simulink model "full_observer"  (R2020b)
settings: Solver=FixedStepAuto  StartTime=0.0  StopTime=20  FixedStep=0.01  RelTol=1e-3
values from neighbouring files (symbols this model uses):
  G = -J_RH*(M_M*L/2+M*l)*(J_RH+N^2*J_m+j)*g    (= -0.22537747671)    [aaaaaaaaaaaaaaaaaaaaaaaaa.m]    (also in disturb_estimation.m = -0.0465293382657; full_obs2.m = -0.0465293382657; fuulll_feedback.m = -0.0465293382657; reduced_observre_2.m = -0.0465293382657)
  H = -N*K_m*J_RH    (= -0.00759948)    [aaaaaaaaaaaaaaaaaaaaaaaaa.m]    (also in disturb_estimation.m = -0.00486576; full_obs2.m = -0.00486576; fuulll_feedback.m = -0.00486576; reduced_observre_2.m = -0.00486576)
  k1 = K(1)    [disturb_estimation.m]    (also in full_obs2.m; fuulll_feedback.m; reduced_observre_2.m)
  k2 = K(2)    [disturb_estimation.m]    (also in full_obs2.m; fuulll_feedback.m; reduced_observre_2.m)
  k3 = K(3)    [disturb_estimation.m]    (also in full_obs2.m; fuulll_feedback.m; reduced_observre_2.m)
  k4 = K(4)    [disturb_estimation.m]    (also in full_obs2.m; fuulll_feedback.m; reduced_observre_2.m)
  K_m = 0.0109    [aaaaaaaaaaaaaaaaaaaaaaaaa.m]    (also in disturb_estimation.m; full_obs2.m; fuulll_feedback.m; reduced_observre_2.m)
  l1 = L(1)    [disturb_estimation.m]    (also in full (2).m = 0.06; full_obs2.m)
  l2 = L(2)    [disturb_estimation.m]    (also in full (2).m = 0.6329; full_obs2.m)
  l3 = L(3)    [disturb_estimation.m]    (also in full (2).m = 0.3; full_obs2.m)
  l4 = L(4)    [disturb_estimation.m]    (also in full (2).m = 0.0875; full_obs2.m)
  l5 = L(5)    [disturb_estimation.m]    (also in full (2).m = 0.0254; full_obs2.m)
  L_m = 0.145    [aaaaaaaaaaaaaaaaaaaaaaaaa.m]    (also in disturb_estimation.m; full_obs2.m; fuulll_feedback.m; reduced_observre_2.m)
  N = 14    [aaaaaaaaaaaaaaaaaaaaaaaaa.m]    (also in disturb_estimation.m = 3; full (2).m = -1.06605676; full_obs2.m = 3; fuulll_feedback.m = 3)
  R_m = 1.6    [aaaaaaaaaaaaaaaaaaaaaaaaa.m]    (also in disturb_estimation.m; full_obs2.m; fuulll_feedback.m; reduced_observre_2.m)
  T = (M_M*L/2+M*l)*(J_RH+N^2*J_m+j)*g    (= 4.52565214276)    [aaaaaaaaaaaaaaaaaaaaaaaaa.m]    (also in disturb_estimation.m = 0.312697165764; full (2).m = [T1;T2;T3;T4;T5;T6;T7]; full_obs2.m = 0.312697165764; fuulll_feedback.m = 0.312697165764)
  W = (J_M+M*l^2)*(J_RH+N^2*J_m+j)-(J_RH)^2    (= 0.0397505665657)    [aaaaaaaaaaaaaaaaaaaaaaaaa.m]    (also in disturb_estimation.m = -0.0192235420783; full (2).m = blkdiag(W_1,W_2,W_3,W_4,W_5,W_6,W_7); full_obs2.m = -0.0192235420783; fuulll_feedback.m = -0.0192235420783)
  Z = (J_M+M*l^2)*(J_RH+N^2*J_m+j)^2-J_RH^2*(J_RH+N^2*J_m+j)    (= 0.251295170273)    [aaaaaaaaaaaaaaaaaaaaaaaaa.m]    (also in disturb_estimation.m = -0.00839686182665; full_obs2.m = -0.00839686182665; fuulll_feedback.m = -0.00839686182665; reduced_observre_2.m = -0.00839686182665)
settings Model: Creator=A family  LastModifiedBy=A family

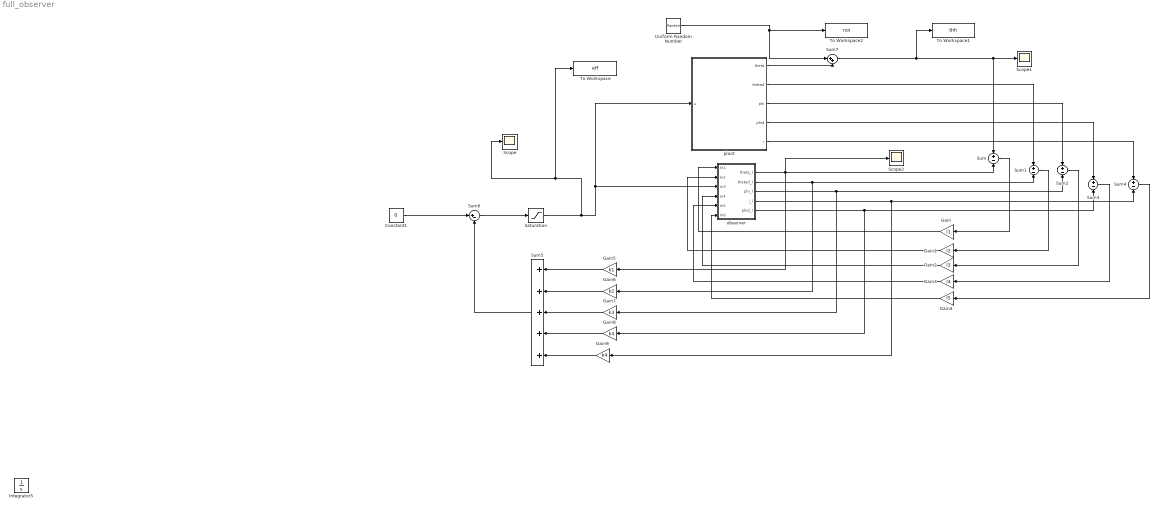
== system full_observer ==
  Constant1 : Constant  Value=0
  Gain : Gain  Gain=l1
  Gain1 : Gain  Gain=l2
  Gain2 : Gain  Gain=l3
  Gain3 : Gain  Gain=l4
  Gain4 : Gain  Gain=l5
  Gain5 : Gain  Gain=k1
  Gain6 : Gain  Gain=k2
  Gain7 : Gain  Gain=k3
  Gain8 : Gain  Gain=k4
  Gain9 : Gain  Gain=k4
  Integrator5 : Integrator
  Saturation : Saturate  UpperLimit=6  LowerLimit=-6
  Scope : Scope
  Scope1 : Scope
  Scope2 : Scope
  Sum{,1..4} (5 alike) : Sum  Inputs=+-
  Sum5 : Sum  Inputs=+++++
  Sum6 : Sum  Inputs=|+-
  Sum7 : Sum  Inputs=|++
  To Workspace : ToWorkspace  VariableName=eff  SampleTime=-1
  To Workspace1 : ToWorkspace  VariableName=thh  SampleTime=-1
  To Workspace2 : ToWorkspace  VariableName=noi  SampleTime=-1
  Uniform Random Number : UniformRandomNumber  Minimum=-0.1  Maximum=0.1  SampleTime=0.01
  observer : Subsystem
  plant : Subsystem
  wires:
  plant/2(thetad) -> Sum1/1
  plant/3(phi) -> Sum2/1
  plant/4(phid) -> Sum3/1
  plant/5(i) -> Sum4/1
  Sum/1 -> Gain/1
  Sum1/1 -> Gain1/1
  Sum2/1 -> Gain2/1
  Sum3/1 -> Gain3/1
  Sum4/1 -> Gain4/1
  Gain/1 -> observer/1(In1)
  Gain1/1 -> observer/2(In2)
  Gain2/1 -> observer/4(In4)
  Gain3/1 -> observer/5(In5)
  Gain4/1 -> observer/6(In6)
  observer/1(theta_l) -> Scope2/1, Gain5/1, Sum/2
  observer/2(thetad_l) -> Gain6/1, Sum1/2
  observer/3(phi_l) -> Gain7/1, Sum2/2
  observer/4(i_l) -> Gain9/1, Sum4/2
  observer/5(phid_l) -> Gain8/1, Sum3/2
  Gain5/1 -> Sum5/1
  Gain6/1 -> Sum5/2
  Gain7/1 -> Sum5/3
  Gain8/1 -> Sum5/4
  Gain9/1 -> Sum5/5
  Sum5/1 -> Sum6/2
  Constant1/1 -> Sum6/1
  Saturation/1 -> To Workspace/1, Scope/1, plant/1(u), observer/3(In3)
  Sum6/1 -> Saturation/1
  Uniform Random Number/1 -> To Workspace2/1, Sum7/1
  plant/1(theta) -> Sum7/2
  Sum7/1 -> To Workspace1/1, Sum/1, Scope1/1

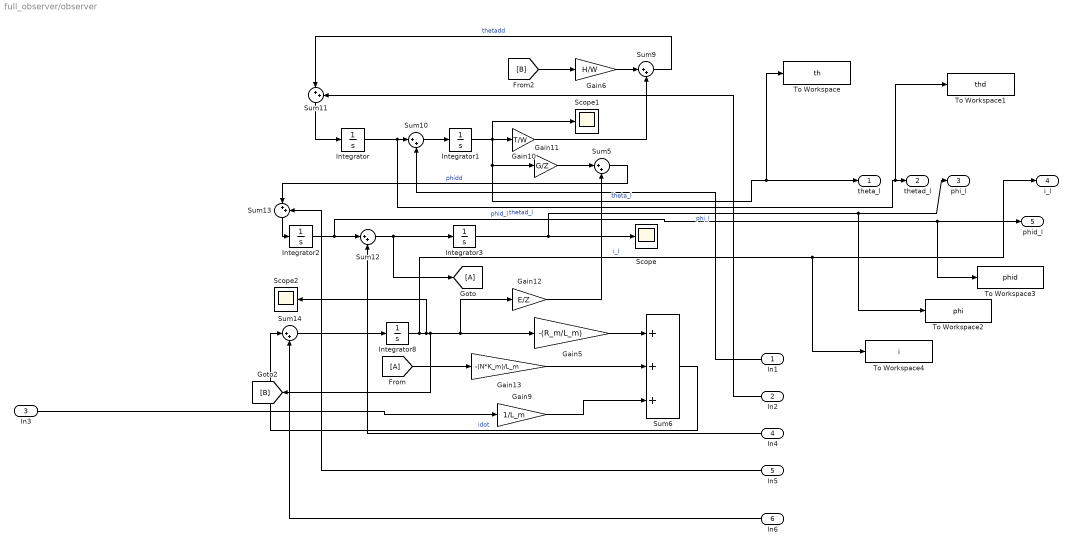
== system full_observer/observer ==
  In1 : Inport
  In2 : Inport  Port=2
  In3 : Inport  Port=3
  In4 : Inport  Port=4
  In5 : Inport  Port=5
  In6 : Inport  Port=6
  Gain10 : Gain  Gain=T/W
  Gain11 : Gain  Gain=G/Z
  Gain12 : Gain  Gain=E/Z
  Gain13 : Gain  Gain=-(N*K_m)/L_m
  Gain5 : Gain  Gain=-(R_m/L_m)
  Gain6 : Gain  Gain=H/W
  Gain9 : Gain  Gain=1/L_m
  Integrator{,1..3,8} (5 alike) : Integrator
  Scope : Scope
  Scope1 : Scope
  Scope2 : Scope
  Sum{5,9..14} (7 alike) : Sum  Inputs=|++
  Sum6 : Sum  Inputs=+++
  To Workspace : ToWorkspace  VariableName=th  SampleTime=-1
  To Workspace1 : ToWorkspace  VariableName=thd  SampleTime=-1
  To Workspace2 : ToWorkspace  VariableName=phi  SampleTime=-1
  To Workspace3 : ToWorkspace  VariableName=phid  SampleTime=-1
  To Workspace4 : ToWorkspace  VariableName=i  SampleTime=-1
  theta_l : Outport
  thetad_l : Outport  Port=2
  phi_l : Outport  Port=3
  i_l : Outport  Port=4
  phid_l : Outport  Port=5
  wires:
  Integrator1/1 -> Scope1/1, theta_l/1, To Workspace/1, Gain11/1, Gain10/1  "theta_l"
  In2/1 -> Sum11/2
  Sum6/1 -> Sum14/1  "idot"
  Sum14/1 -> Integrator8/1
  Sum10/1 -> Integrator1/1
  Sum11/1 -> Integrator/1
  Sum12/1 -> [A], Integrator3/1
  Gain5/1 -> Sum6/1
  Gain6/1 -> Sum9/1
  Sum13/1 -> Integrator2/1
  Sum9/1 -> Sum11/1  "thetadd"
  Sum5/1 -> Sum13/1  "phidd"
  Integrator/1 -> To Workspace1/1, thetad_l/1, Sum10/1  "thetad_l"
  Gain10/1 -> Sum9/2
  Integrator8/1 -> To Workspace4/1, i_l/1, Gain5/1, Gain12/1, [B], Scope2/1  "i_l"
  In5/1 -> Sum13/2
  Integrator2/1 -> To Workspace3/1, phid_l/1, Sum12/1  "phid_l"
  [A] -> Gain13/1
  In4/1 -> Sum12/2
  In3/1 -> Gain9/1
  Gain13/1 -> Sum6/2
  Gain12/1 -> Sum5/2
  Integrator3/1 -> To Workspace2/1, phi_l/1, Scope/1  "phi_l"
  [B] -> Gain6/1
  Gain11/1 -> Sum5/1
  Gain9/1 -> Sum6/3
  In6/1 -> Sum14/2
  In1/1 -> Sum10/2

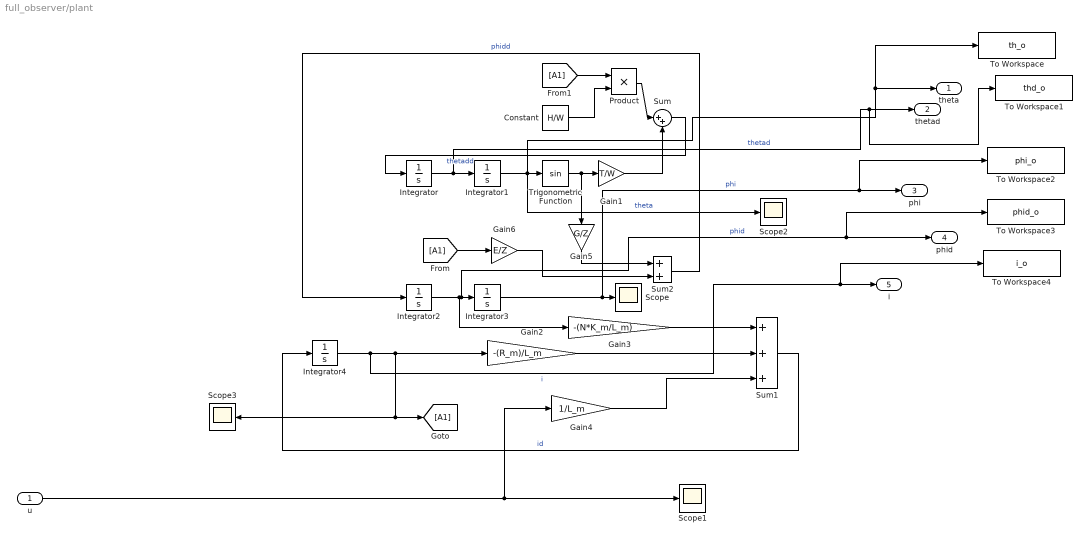
== system full_observer/plant ==
  u : Inport
  Constant : Constant  Value=H/W
  Gain1 : Gain  Gain=T/W
  Gain2 : Gain  Gain=-(R_m)/L_m
  Gain3 : Gain  Gain=-(N*K_m/L_m)
  Gain4 : Gain  Gain=1/L_m
  Gain5 : Gain  Gain=G/Z
  Gain6 : Gain  Gain=E/Z
  Integrator{,2..4} (4 alike) : Integrator
  Integrator1 : Integrator  InitialCondition=20*pi/180
  Product : Product
  Scope{,1..3} (4 alike) : Scope
  Sum : Sum  Inputs=|++
  Sum1 : Sum  Inputs=+++
  Sum2 : Sum
  To Workspace : ToWorkspace  VariableName=th_o  SampleTime=-1
  To Workspace1 : ToWorkspace  VariableName=thd_o  SampleTime=-1
  To Workspace2 : ToWorkspace  VariableName=phi_o  SampleTime=-1
  To Workspace3 : ToWorkspace  VariableName=phid_o  SampleTime=-1
  To Workspace4 : ToWorkspace  VariableName=i_o  SampleTime=-1
  Trigonometric Function : Trigonometry
  theta : Outport
  thetad : Outport  Port=2
  phi : Outport  Port=3
  phid : Outport  Port=4
  i : Outport  Port=5
  wires:
  Integrator/1 -> To Workspace1/1, thetad/1, Integrator1/1  "thetad"
  Integrator2/1 -> To Workspace3/1, phid/1, Integrator3/1, Gain3/1  "phid"
  Integrator4/1 -> Gain2/1, Scope3/1, [A1], To Workspace4/1, i/1  "i"
  Gain5/1 -> Sum2/1
  u/1 -> Scope1/1, Gain4/1
  Product/1 -> Sum/1
  Sum2/1 -> Integrator2/1  "phidd"
  Integrator1/1 -> To Workspace/1, theta/1, Scope2/1, Trigonometric Function/1  "theta"
  Gain4/1 -> Sum1/3
  Integrator3/1 -> To Workspace2/1, phi/1, Scope/1  "phi"
  [A1] -> Gain6/1
  Gain6/1 -> Sum2/2
  [A1] -> Product/1
  Constant/1 -> Product/2
  Gain1/1 -> Sum/2
  Trigonometric Function/1 -> Gain5/1, Gain1/1
  Gain3/1 -> Sum1/1
  Gain2/1 -> Sum1/2
  Sum1/1 -> Integrator4/1  "id"
  Sum/1 -> Integrator/1  "thetadd"
